simulink model "sim_validation_3DoF"  (R2024b)
settings: Solver=VariableStepAuto  StartTime=0.0  StopTime=tf  RelTol=1e-12  AbsTol=1e-12
values from neighbouring files (symbols this model uses):
  alpha = 0.5086    [3DoF_deterministic_Workspace.mat]    (also in Compressed_Time_Step_2dof_Experiment.mat; Copy_of_Deterministic_6DoF.m; Copy_of_Deterministic_6DoF_quat.m; Copy_of_SCP_Earth_Mars_transfer_GA_uniform_adaptive.m = 1)
  I = 0.15    [3DoF_deterministic_Workspace.mat]    (also in Copy_of_DQG_6DoF_fixedtf.m = [4.2; 4.2; 0.6]; Copy_of_Deterministic_6DoF.m = [50000; 150000; 150000] * (1e-3) ^ 2; Copy_of_Deterministic_6DoF_quat.m = [50000; 150000; 150000] * (1e-3) ^ 2; DQG_6DoF.m = [4.2; 4.2; 0.6])
  input_vector = 1:nu    [Deterministic_3DoF_with_mass_convexified_reynolds.m]    (also in Deterministic_3DoF_with_mass_convexified_takeoffdivert.m; Deterministic_3DoF_with_mass_polar.m; Deterministic_6DoF.m; Deterministic_6DoF_reynolds.m)
  L = 0.003    [3DoF_deterministic_Workspace.mat]    (also in Compressed_Time_Step_2dof_Experiment.mat; Copy_of_DQG_6DoF_fixedtf.m = 1; Copy_of_Deterministic_6DoF.m; Copy_of_Deterministic_6DoF_quat.m)
  m_0 = 2100    [3DoF_deterministic_Workspace.mat]    (also in Compressed_Time_Step_2dof_Experiment.mat = 2000; Copy_of_Deterministic_6DoF.m = 2600; Copy_of_Deterministic_6DoF_quat.m = 2600; Copy_of_SCP_Earth_Mars_transfer_GA_uniform_adaptive.m = 1)
  r_0 = [0 4.6]    [3DoF_deterministic_Workspace.mat]    (also in Compressed_Time_Step_2dof_Experiment.mat = [1 1.5]; Copy_of_Deterministic_6DoF.m = [0.5; -0.2; 2.0]; Copy_of_Deterministic_6DoF_quat.m = [0.5; -0.2; 2.0]; Deterministic_2DoF_linear.m = [0; 4.6])
  state_vector = 1:nx    [Deterministic_3DoF_with_mass_convexified_reynolds.m]    (also in Deterministic_3DoF_with_mass_convexified_takeoffdivert.m; Deterministic_3DoF_with_mass_polar.m; Deterministic_6DoF.m; Deterministic_6DoF_reynolds.m)
  v_0_b = make_R2(theta_0)' * v_0 - eye(2, 3) * cross([0; 0; w_0], [r_0; 0])    [Deterministic_3DoF_with_mass_convexified_reynolds.m]    (also in Deterministic_3DoF_with_mass_convexified_takeoffdivert.m; Deterministic_3DoF_with_mass_polar.m; Deterministic_6DoF.m = angle2dcm(theta1_0, theta2_0, theta3_0, "XYX") * v_0; Deterministic_6DoF_reynolds.m = angle2dcm(theta1_0, theta2_0, theta3_0, "XYX") * v_0)
  x_0 = [0 4.6 0.153 -0.265003773558 2.09439510239 0 2100]    [3DoF_deterministic_Workspace.mat]    (also in Compressed_Time_Step_2dof_Experiment.mat = [1 1.5 0 0 7.60090245954]; Copy_of_DQG_6DoF_fixedtf.m = [m_i; construct_dual_quat(q_i, r_I_i); w_B_i; quat_rot(q_i, ; Copy_of_Deterministic_6DoF.m = [r_0; v_0; theta_0; w_0]; Copy_of_Deterministic_6DoF_quat.m = [r_0; v_0; q_0; w_0])
libraries: aerolibanim x1, simulink_extras x1, aerolibanimutils x1
settings Model: Creator=thatf  LastModifiedBy=thatf

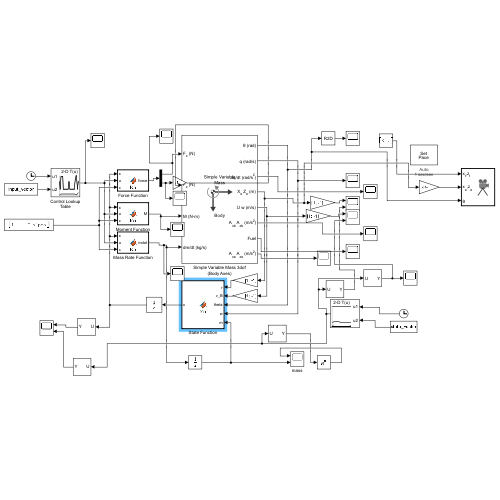
[thumbnail: Simulink's stored preview of the top-level diagram]
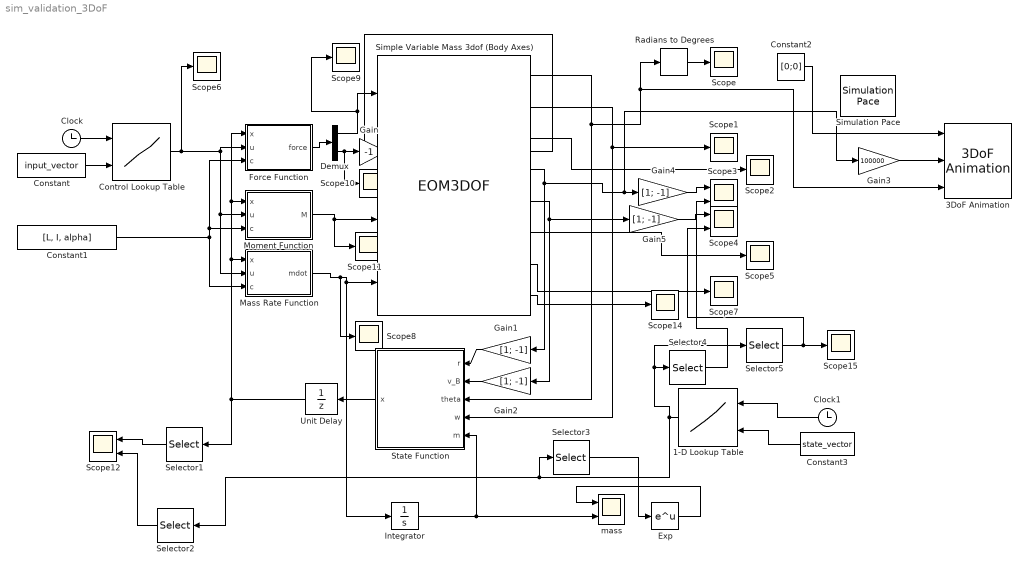
== system sim_validation_3DoF ==
  1-D Lookup Table : Lookup_n-D  BreakpointsForDimension1=opt_time'  BreakpointsForDimension2=state_vector  Table=x_opt'  InternalRulePriority=Speed  RndMeth=Simplest
      settings: InputPortMap=u0,u1
  3DoF Animation : aerolibanim/3DoF Animation  u1=[-1000 1000 -100 100 -5000 50]  u2=0.05  u3=2.0  u5=Fly alongside  u6=[0 1000 0]  u7=80  u8=on
  Clock : Clock
  Clock1 : Clock
  Constant : Constant  Value=input_vector
  Constant1 : Constant  Value=[L, I, alpha]
  Constant2 : Constant  Value=[0;0]
  Constant3 : Constant  Value=state_vector
  Control Lookup Table : Lookup_n-D  BreakpointsForDimension1=opt_time'  BreakpointsForDimension2=input_vector  Table=control_inputs'  InternalRulePriority=Speed  RndMeth=Simplest
      settings: InputPortMap=u0,u1
  Demux : Demux  Outputs=2
  Exp : Math
  Force Function : MATLAB Function  TreatAsAtomicUnit=on
  Gain : Gain  Gain=-1
  Gain{1..2,4..5} (4 alike) : Gain  Gain=[1; -1]
  Gain3 : Gain  Gain=100000
  Integrator : Integrator  InitialCondition=m_0
  Mass Rate Function : MATLAB Function  TreatAsAtomicUnit=on
  Moment Function : MATLAB Function  TreatAsAtomicUnit=on
  Radians to Degrees : simulink_extras/Transformations/Radians to Degrees
  Scope{,1..2,5..11,14..15} (12 alike) : Scope
  Scope12 : Scope  NumInputPorts=2
  Scope3 : Scope  NumInputPorts=2
  Scope4 : Scope  NumInputPorts=2
  Selector1 : Selector  InputPortWidth=7  IndexOptions=Index vector (dialog)  Indices=[5]  OutputSizes=1
  Selector2 : Selector  InputPortWidth=7  IndexOptions=Index vector (dialog)  Indices=[5]  OutputSizes=1
  Selector3 : Selector  InputPortWidth=7  IndexOptions=Index vector (dialog)  Indices=[7]  OutputSizes=1
  Selector4 : Selector  InputPortWidth=7  IndexOptions=Index vector (dialog)  Indices=[1,2]  OutputSizes=1
  Selector5 : Selector  InputPortWidth=7  IndexOptions=Index vector (dialog)  Indices=[3,4]  OutputSizes=1
  Simple Variable Mass 3dof (Body Axes) : EOM3DOF  mtype=Simple Variable  v_ini=norm(v_0_b .* [1; -1])  theta_ini=theta_0  q_ini=w_0  alpha_ini=incidence_0  pos_ini=r_0 .* [1; -1]  mass=m_0  mass_e=m_dry  mass_f=m_0  Iyy_e=I - 1e-12  Iyy_f=I  g=9.81e-3  abi_flag=on
  Simulation Pace : aerolibanimutils/Simulation Pace  SimulationPace=1  SleepMode=Auto  OutputPaceError=off  SampleTime=1/30
  State Function : MATLAB Function  TreatAsAtomicUnit=on
  Unit Delay : UnitDelay  InitialCondition=x_0  SampleTime=-1  HasFrameUpgradeWarning=on
  mass : Scope  NumInputPorts=2
  wires:
  Clock/1 -> Control Lookup Table/1
  Control Lookup Table/1 -> Scope6/1, Force Function/2(u), Mass Rate Function/2(u), Moment Function/2(u)
  Moment Function/1(M) -> Scope11/1, Simple Variable Mass 3dof (Body Axes)/3
  Mass Rate Function/1(mdot) -> Scope8/1, Simple Variable Mass 3dof (Body Axes)/4, Integrator/1
  Simple Variable Mass 3dof (Body Axes)/3 -> Scope2/1
  Simple Variable Mass 3dof (Body Axes)/4 -> Gain1/1, Gain3/1, Gain4/1
  Simple Variable Mass 3dof (Body Axes)/5 -> Gain5/1, Gain2/1
  Simple Variable Mass 3dof (Body Axes)/6 -> Scope5/1
  Simple Variable Mass 3dof (Body Axes)/7 -> Scope7/1
  Force Function/1(force) -> Demux/1
  Demux/2 -> Scope10/1, Gain/1
  Demux/1 -> Scope9/1, Simple Variable Mass 3dof (Body Axes)/1
  Constant/1 -> Control Lookup Table/2
  Constant1/1 -> Force Function/3(c), Moment Function/3(c), Mass Rate Function/3(c)
  Gain1/1 -> State Function/1(r)
  Gain2/1 -> State Function/2(v_B)
  State Function/1(x) -> Unit Delay/1
  Unit Delay/1 -> Selector1/1, Force Function/1(x), Moment Function/1(x), Mass Rate Function/1(x)
  Constant2/1 -> 3DoF Animation/1
  Radians to Degrees/1 -> Scope/1
  Gain3/1 -> 3DoF Animation/2
  Gain4/1 -> Scope3/1
  Integrator/1 -> State Function/5(m), mass/2
  Clock1/1 -> 1-D Lookup Table/1
  Constant3/1 -> 1-D Lookup Table/2
  Simple Variable Mass 3dof (Body Axes)/2 -> State Function/4(w), Scope1/1
  1-D Lookup Table/1 -> Selector5/1, Selector4/1, Selector3/1, Selector2/1
  Selector1/1 -> Scope12/1
  Selector2/1 -> Scope12/2
  Simple Variable Mass 3dof (Body Axes)/1 -> State Function/3(theta), 3DoF Animation/3, Radians to Degrees/1
  Gain/1 -> Simple Variable Mass 3dof (Body Axes)/2
  Simple Variable Mass 3dof (Body Axes)/8 -> Scope14/1
  Gain5/1 -> Scope4/1
  Selector3/1 -> Exp/1
  Exp/1 -> mass/1
  Selector4/1 -> Scope3/2
  Selector5/1 -> Scope15/1, Scope4/2

== matlab function sim_validation_3DoF/Moment Function ==
  data: x input; u input; M output; c input
function M = fcn(x, u, c)
% 
% thrust_mag = u(1);
% gimbal = u(2);
% L = c(1);
% 
% T = thrust_mag * [cos(gimbal); sin(gimbal)];
% 
% M = [0, 0, 1] * cross([-L; 0; 0], [T; 0]);


m = exp(x(7));
a = u(1:2);
L = c(1);

T = m * a;

M = [0, 0, 1] * cross([-L; 0; 0], [T; 0]);

== matlab function sim_validation_3DoF/Force Function ==
  data: x input; u input; force output; c input
function force = fcn(x, u, c)
% thrust_mag = u(1);
% gimbal = u(2);
% 
% force = thrust_mag * [cos(gimbal); sin(gimbal)];

m = exp(x(7));
a = u(1:2);

force = m * a;

== matlab function sim_validation_3DoF/Mass Rate Function ==
  data: x input; u input; mdot output; c input
function mdot = fcn(x, u, c)

% thrust_mag = u(1);
% 
% alpha = c(3);
% 
% mdot = -alpha * thrust_mag;
% 

m = exp(x(7));
a = norm(u(1:2));

T = a * m;

alpha = c(3);

mdot = -alpha * T;

== matlab function sim_validation_3DoF/State Function ==
  data: r input; x output; v_B input; theta input; w input; m input
function x = fcn(r, v_B, theta, w, m)

v = make_R2(theta) * (v_B + eye(2, 3) * cross([0; 0; w], [v_B; 0]));

x = [r; v; theta; w; log(m)];
